simulink model "CONTROL"  (R2022a)
settings: Solver=FixedStepAuto  StartTime=0.0  StopTime=inf  FixedStep=ts  RelTol=1e-3
values from neighbouring files (symbols this model uses):
  ts = 1e-2    (= 0.01)    [init.m]    (also in params.mat)
libraries: instrumentseriallib x2
settings Model: Creator=Ponchito  LastModifiedBy=Ponchito

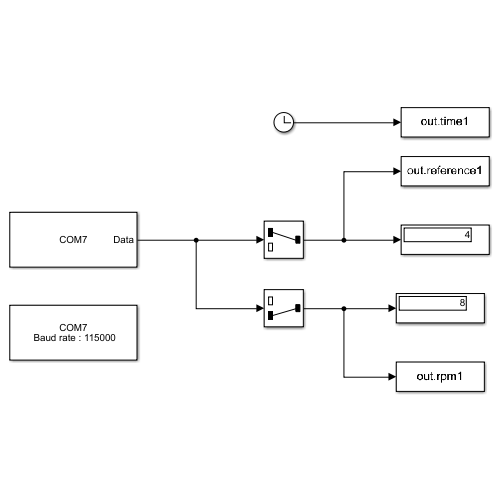
[thumbnail: Simulink's stored preview of the top-level diagram]
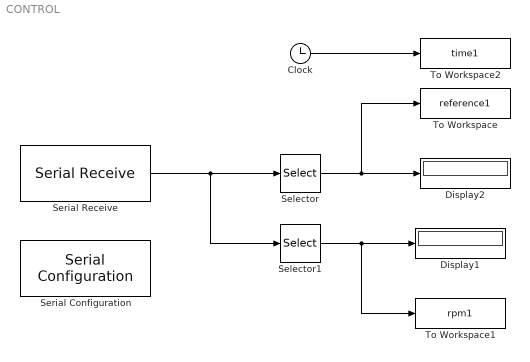
== system CONTROL ==
  Clock : Clock
  Display1 : Display
  Display2 : Display
  Selector : Selector  InputPortWidth=2  IndexOptions=Index vector (dialog)  Indices=[1]  OutputSizes=1
  Selector1 : Selector  InputPortWidth=2  IndexOptions=Index vector (dialog)  Indices=[2]  OutputSizes=1
  Serial Configuration : instrumentseriallib/Serial Configuration  Priority=-200000  PortSel=COM7  Port=COM7  ComPort=COM7  BaudRate=115000  DataBits=8  Parity=none  StopBits=1  ByteOrder=little-endian  FlowControl=none  Timeout=10  SimulateUsing=Interpreted execution  BlockInModel=on  aMode=1
      settings: SourceProductBaseCode=OT,IC,MT
  Serial Receive : instrumentseriallib/Serial Receive  Priority=1  PortSel=COM7  Port=COM7  ComPort=COM7  DataType=uint16  SaveDataType=uint8  ToggleHeader=off  Header=[]  ToggleTerminator=off  Terminator=<none>  CustomTerminator=[]  InputFormat=Column major  ToggleDataSize=on  DataSize=[1 2]  EnableBlockingMode=on  ActionDataUnavailable=Output last received value  ActionWhenDataUnavailable=Output last received value  CustomValue=0  SampleTime=ts  SimulateUsing=Interpreted execution  BlockInModel=on  aMode=1
      settings: SourceProductBaseCode=OT,IC,MT
  To Workspace : ToWorkspace  VariableName=reference1  SampleTime=-1
  To Workspace1 : ToWorkspace  VariableName=rpm1  SampleTime=-1
  To Workspace2 : ToWorkspace  VariableName=time1  SampleTime=-1
  wires:
  Selector/1 -> Display2/1, To Workspace/1
  Selector1/1 -> To Workspace1/1, Display1/1
  Serial Receive/1 -> Selector1/1, Selector/1
  Clock/1 -> To Workspace2/1
